simulink model "WholeBloodTEGModel_6P_B"  (R2021a)
settings: Solver=VariableStepAuto  StartTime=0.0  StopTime=75  RelTol=1e-3
model workspace (MAT data in the model file):
  SDO_OutputTimes = [0 0.0833333333333 0.166666666667 0.25 0.333333333333 0.416666666667 0.5 0.583333333333 0.666666666667 0.75 0.833333333333 0.916666666667 ... (901 elements, 901x1)]
values from neighbouring files (symbols this model uses):
  Kd1 = 2    [TEG_WB_6Param_SDO_Fit.m]    (also in TEG_WB_Trauma_Visualization.m = WB_Fit_Par(i,3); WholeBloodTEGModel3piece_Fits_setup_Save.m)
  Kd2 = 35    [TEG_WB_6Param_SDO_Fit.m]    (also in TEG_WB_Trauma_Visualization.m = WB_Fit_Par(i,5); WholeBloodTEGModel3piece_Fits_setup_Save.m = 30)
  Kn1 = 2.5e10    (= 25000000000)    [TEG_WB_6Param_SDO_Fit.m]    (also in TEG_WB_Trauma_Visualization.m = WB_Fit_Par(i,1); WholeBloodTEGModel3piece_Fits_setup_Save.m = 5000000000)
  Kn2 = 2.5e10    (= 25000000000)    [TEG_WB_6Param_SDO_Fit.m]    (also in TEG_WB_Trauma_Visualization.m = WB_Fit_Par(i,4); WholeBloodTEGModel3piece_Fits_setup_Save.m = 50000000)
  Kp1 = 5    [TEG_WB_6Param_SDO_Fit.m]    (also in TEG_WB_Trauma_Visualization.m = WB_Fit_Par(i,2); WholeBloodTEGModel3piece_Fits_setup_Save.m = 0.2)
  Kp2 = 5    [TEG_WB_6Param_SDO_Fit.m]
settings Model: OrderedModelArguments=off  Creator=m.perezblanco  LastModifiedBy=s.ghetmiri
settings SolverCC: AlgebraicLoopSolver=TrustRegion
settings DataIOCC: ExternalInput=tp8c430dcf_48af_4c60_b80f_fc1e10a15a6b(1)  LoadExternalInput=on  OutputOption=AdditionalOutputTimes  OutputTimes=SDO_OutputTimes  ReturnWorkspaceOutputsName=SDOSimTest_Log
settings DebuggingCC: SFMachineParentedDataDiag=warning  ArithmeticOperatorsInVariantConditions=warning
settings SFSimCC: SimUseLocalCustomCode=off  CustomCodeUndefinedFunction=UseInterfaceOnly
settings RTWCC: RTWUseLocalCustomCode=off

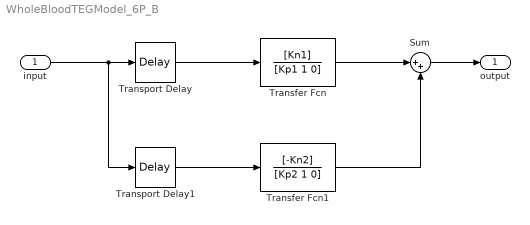
== system WholeBloodTEGModel_6P_B ==
  input : Inport
  Sum : Sum  Inputs=|++
  Transfer Fcn : TransferFcn  Numerator=[Kn1]  Denominator=[Kp1 1 0]
  Transfer Fcn1 : TransferFcn  Numerator=[-Kn2]  Denominator=[Kp2 1 0]
  Transport Delay : TransportDelay  DelayTime=Kd1
  Transport Delay1 : TransportDelay  DelayTime=Kd2
  output : Outport  SignalName=y  VectorParamsAs1DForOutWhenUnconnected=off
  wires:
  input/1 -> Transport Delay1/1, Transport Delay/1
  Transport Delay/1 -> Transfer Fcn/1
  Sum/1 -> output/1
  Transfer Fcn/1 -> Sum/1
  Transfer Fcn1/1 -> Sum/2
  Transport Delay1/1 -> Transfer Fcn1/1
